simulink library "LevelDetectorLibBtc"  (R2022b)
settings: Solver=VariableStepAuto  StartTime=0.0  StopTime=10.0  RelTol=1e-3
values from neighbouring files (symbols this model uses):
  AnnTriggerThreshold = single(0.5)    [LevelDetectorConfig.m]
  SuperFastDecayMultiplier = single(3.0)    [LevelDetectorConfig.m]
libraries: HandyTextFile x1
settings Model: Creator=kl13806  LastModifiedBy=kl13806
settings SolverCC: AlgebraicLoopSolver=TrustRegion
settings DebuggingCC: UnconnectedInputMsg=warning  UnconnectedOutputMsg=warning  UnconnectedLineMsg=warning  SFMachineParentedDataDiag=warning
settings ModelReferenceCC: EnableRefExpFcnMdlSchedulingChecks=on
settings RTWCC: DLArmComputeVersion=19.05

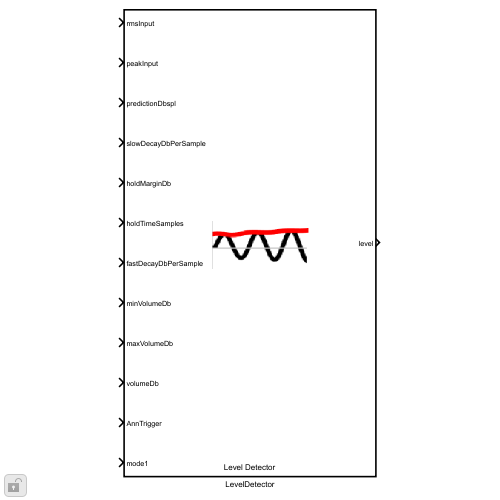
[thumbnail: Simulink's stored preview of the top-level diagram]
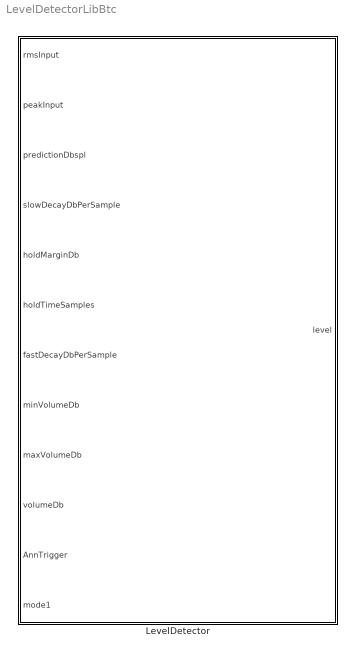
== system LevelDetectorLibBtc ==
  LevelDetector : MATLAB Function  TreatAsAtomicUnit=on  mask(Blocklib LevelDetector){Config=[]}
      mask prompts: Config "LevelDetectorConfig"
      mask help: Computes signal level in dB using a combination of the attack, slow decay, hold and fast decay phases. Check the Help menu for a description of the parameters.
      mask init:
      | blkh=gcbh;
      | Config=BTConfig.Assert(blkh,Config);
      | Config.Validate();
      | 
      | % Flatten Config properties for use by MFB...
      | % which is immediately under this mask (no subsystem)
      | BTConfig.Expand(Config);

== matlab function LevelDetectorLibBtc/LevelDetector ==
  data: rmsInput input; peakInput input; predictionDbspl input; slowDecayDbPerSample input; holdMarginDb input; holdTimeSamples input; fastDecayDbPerSample input; minVolumeDb input; maxVolumeDb input; volumeDb input; AnnTrigger input; level output; mode1 input; AnnTriggerThreshold parameter; SuperFastDecayMultiplier parameter
function level = levelDetector(rmsInput, peakInput, predictionDbspl, ...
    slowDecayDbPerSample, holdMarginDb, holdTimeSamples, fastDecayDbPerSample, ...
    minVolumeDb, maxVolumeDb, volumeDb, AnnTrigger, mode1, ... % inputs
    AnnTriggerThreshold, SuperFastDecayMultiplier) % parameters
   
    % States
    persistent holdFlag;
    persistent holdState;
    persistent envelope1;

    if (isempty(holdFlag))
        holdFlag = 1;
        holdState = 0;
        envelope1 = -abs(minVolumeDb);
    end

    % By default we use the RMS input
    input1 = rmsInput;
    level = single(0.0);
    
    if mode1 >= 0.0
        % Choose input1 based on mode1
        if (mode1 > 0.0)
            input1 = peakInput;
        end
        delta = single( envelope1 - input1 );
        if ( delta <= single(0) )
            % Attack phase
            envelope1 = input1;
            holdState = 0;
            holdFlag = 1;
        else
            % Slow Decay phase
            coef = slowDecayDbPerSample;   
            
            % Hold phase
            if ( delta >= holdMarginDb )
                holdState = holdState + 1;
                if ( holdState > holdTimeSamples )
                    holdFlag = 0;
                end
            else                
                holdState = 0;
            end
            
            % Fast decay phase
            if holdFlag == 0
                coef = fastDecayDbPerSample;
            end
            
            % Super fast decay phase
            if ( AnnTrigger > AnnTriggerThreshold )
                coef = SuperFastDecayMultiplier * fastDecayDbPerSample;
            end
            
            % Update the envelope1
            envelope1 = envelope1 + coef;
        end
        % Boundary Check
        envelope1 = max(minVolumeDb, envelope1);
        envelope1 = min(maxVolumeDb, envelope1);
        
        % dBSPL Conversion
        level = max(0, envelope1 + predictionDbspl + volumeDb);
    end
end

    % Description: 
    % Based on the difference between the envelope1 and the input, we
    % decide whether to go into the attack, slow decay or hold phases.
    
    % If the input is greater than the envelope1, we attack immediately and 
    % reset the Hold counter to get ready for a possible Hold phase. The 
    % Hold flag indicates whether or not the Hold phase is done (0 when done).
    
    % Otherwise, we enter the decay phases. 
    % If delta is within the hold margin => input is not decreasing 
    % "drastically", slow decay coefficient is applied but the Hold counter
    % is not incremented. If greater than the hold margin, we want to make 
    % sure that it is not a "sudden" dip, hence we "hold" the level, i.e. 
    % increment a Hold counter, while applying the same slow decay coefficient.     
    % At any point in the Hold phase, if delta goes lower than the hold 
    % margin we reset the counter and get out of the Hold phase.
    
    % If the level was "held" for all of the hold time, it means that the 
    % input is indeed dropping and we want to catch up with the input 
    % faster, hence we apply a "fast decay" coefficient.
    % Announcements take precedence over all decay phases.
